simulink model "simu"  (R2025a)
settings: Solver=VariableStepAuto  StartTime=0.0  StopTime=10.0  RelTol=1e-3
settings Model: Creator=JONIK  LastModifiedBy=JONIK

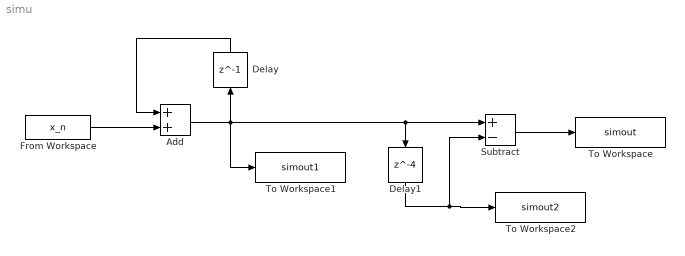
== system simu ==
  Add : Sum  AccumDataTypeStr=uint8
  Delay : Delay  DelayLength=1  InitialCondition=0
  Delay1 : Delay  DelayLength=4  InitialCondition=0
  From Workspace : FromWorkspace  VariableName=x_n  SampleTime=0.0001
  Subtract : Sum  Inputs=+-  AccumDataTypeStr=uint8
  To Workspace : ToWorkspace  VariableName=simout  SaveFormat=Timeseries  SampleTime=-1
  To Workspace1 : ToWorkspace  VariableName=simout1  SaveFormat=Timeseries  SampleTime=-1
  To Workspace2 : ToWorkspace  VariableName=simout2  SaveFormat=Timeseries  SampleTime=-1
  wires:
  From Workspace/1 -> Add/2
  Add/1 -> To Workspace1/1, Delay/1, Delay1/1, Subtract/1
  Delay/1 -> Add/1
  Subtract/1 -> To Workspace/1
  Delay1/1 -> To Workspace2/1, Subtract/2
